simulink model "forces_cosimulation"  (R2021b)
settings: Solver=ode45  StartTime=0.0  StopTime=40  FixedStep=0.01  RelTol=1e-3  EnableMultiTasking=on
libraries: instrumentlib x2, simulink x2
settings Model: PacingRate=11  Creator=tasora  LastModifiedBy=Trevor
settings SolverCC: AlgebraicLoopSolver=TrustRegion
settings DataIOCC: LimitDataPoints=on  SaveFormat=Array  SignalLoggingSaveFormat=ModelDataLogs  ReturnWorkspaceOutputs=off
settings OptimizationCC: ExpressionDepthLimit=2147483647  LifeSpan=inf
settings DebuggingCC: UnderspecifiedInitializationDetection=Classic  MergeDetectMultiDrivingBlocksExec=none  SolverPrmCheckMsg=warning  FcnCallInpInsideContextMsg=warning  StateNameClashWarn=warning  SFUnexpectedBacktrackingDiag=warning  SFNoUnconditionalDefaultTransitionDiag=warning  SFExecutionAtInitializationDiag=none  SFMachineParentedDataDiag=warning  ArithmeticOperatorsInVariantConditions=warning
settings HardwareCC: ProdBitPerPointer=32  ProdBitPerSizeT=32  ProdBitPerPtrDiffT=32  ProdLargestAtomicFloat=None  ProdIntDivRoundTo=Undefined  ProdEndianess=Unspecified  ProdWordSize=32  ProdHWDeviceType=32-bit Generic
settings ModelReferenceCC: PropagateSignalLabelsOutOfModel=off
settings SFSimCC: SimUseLocalCustomCode=off  CustomCodeUndefinedFunction=UseInterfaceOnly
settings RTWCC: RTWUseLocalCustomCode=off
settings CodeAppCC: StateflowObjectComments=on
settings GRTTargetCC: TargetLangStandard=C89/C90 (ANSI)  CombineOutputUpdateFcns=off  GRTInterface=on
settings ConfigComp: CovMetricSettings=dw  CovSaveCumulativeToWorkspaceVar=on  CovSaveSingleToWorkspaceVar=on  CovExternalEMLEnable=off

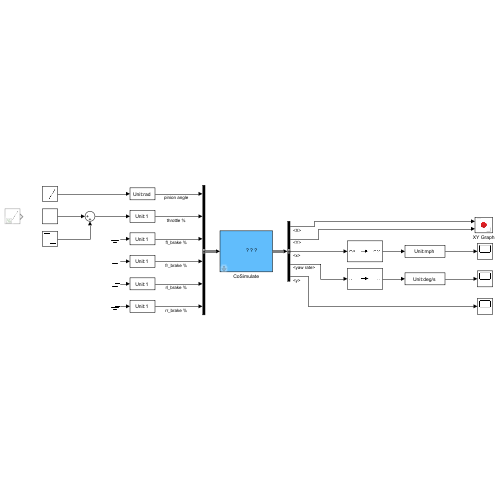
[thumbnail: Simulink's stored preview of the top-level diagram]
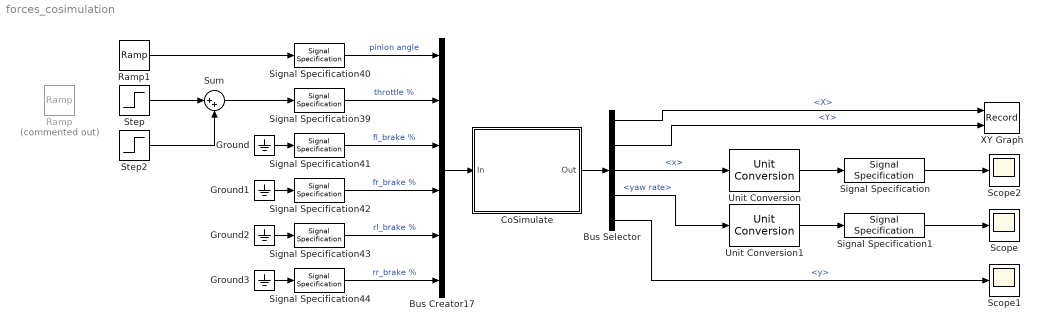
== system forces_cosimulation ==
  Bus Creator17 : BusCreator  Inputs=6
  Bus Selector : BusSelector  OutputSignals=global frame.position.X,global frame.position.Y,chassis frame.velocity.x,chassis frame.rotational velocity.yaw rate,chassis frame.acceleration.y
  CoSimulate : Subsystem  Description=|  mask{com_step=1e-2, tcp_data_size=39, host_name=localhost, tcp_port=50009, tcp_timeout=5}
      | This block can be used to exchange data with Chrono::Engine.                                                                                      
      | A Chrono::Engine program with a running ChCosimulation inferface must be started, it will work as a server; then the Simulink program must be run.
      | Note! check that the dimensions of the exchanged vectors do match!
      mask prompts: com_step "Communication step size"; tcp_data_size "N. of scalars received from C::E (as block output)"; host_name "TCP host name (ex. 'localhost', or 'www.myhost.com')"; tcp_port "TCP port (ex. 50007)"; tcp_timeout "TCP timeout (seconds)"
      mask init:
      | block_receive = [gcb, '/TCP Receive'];
      | set_param(block_receive, 'SampleTime', num2str(com_step));
      | set_param(block_receive, 'Host', host_name);
      | set_param(block_receive, 'Port', num2str(tcp_port));
      | set_param(block_receive, 'DataSize', num2str(tcp_data_size+1));
      | set_param(block_receive, 'Timeout', num2str(tcp_timeout));
      | block_send = [gcb, '/TCP Send'];
      | set_param(block_send, 'Host', host_name);
      | set_param(block_send, 'Port', num2str(tcp_port));
      mask Display:
      | image(imread('block_logo.png'))
      | disp('C::E                   ')
  Ground{,1..3} (4 alike) : Ground
  Ramp : simulink/Sources/Ramp  Commented=on  slope=0.1  start=4  InitialOutput=0
  Ramp1 : simulink/Sources/Ramp  slope=0.01  start=15  InitialOutput=0
  Scope : Scope
  Scope1 : Scope
  Scope2 : Scope
  Signal Specification : SignalSpecification  Unit=mph
  Signal Specification1 : SignalSpecification  Unit=deg/s
  Signal Specification{39,41..44} (5 alike) : SignalSpecification  Unit=1
  Signal Specification40 : SignalSpecification  Unit=rad
  Step : Step  Time=3  After=0.75  SampleTime=0
  Step2 : Step  Time=15  After=-0.05  SampleTime=0
  Sum : Sum  Inputs=|++
  Unit Conversion : UnitConversion
  Unit Conversion1 : UnitConversion
  XY Graph : Record  FileSettingsInternal="{\"entries\":[{\"content\":{\"excelSettings\":{\"content\":{},\"type\":\"Streamout.ExcelSettings\"}},\"type\":\"Streamout.FileSettingStorage\",\"uuid\":\"5bc0685a-b1bb-4583-b74f-d6d04f37d9c6\"}],\"packageUris\":[\"http://schema.mathworks.com/mf0/streamout_blocks/R2020a\"],\"version\":\"1.0\"}"  Layout=[1 1]  SignalsInternal="{\"entries\":[{\"content\":{\"signals\":[{\"content\":{\"blockPath\":[\"forces_cosimulation/XY Graph\"],\"channel\":[],\"dimensions\":[1,1],\"domain\":\"forces_cosimulation/XY Graph\",\"lineColor\":\"#a2142f\",\"plots\":[1],\"port\":1,\"sid\":[\"\"],\"signalID\":3435,\"signalName\":\"<X>\"},\"type\":\"RecordBlkView.Signal\",\"uuid\":\"5aa4ce1d-9ab9-452c-9b58-d05b75f7601c\"},{\"content\":{\"blockPath\":[\"forces_cosimulation/XY Graph\"],\"channel\":[],\"dimensions\":[1,1],\"domain\":\"forces_cosimulation/XY Graph\",\"lineColor\":\"#139fff\",\"plots\":[1],\"port\":2,\"sid\":[\"\"],\"signalID\":3439,\"signalName\":\"<Y>\"},\"type\":\"RecordBlkView.Signal\",\"uuid\":\"38391aed-c002-4d5f-92b2-354e32cfb4eb\"}]},\"type\":\"RecordBlkView.InputSignals\",\"uuid\":\"4796c31f-e78f-4ee8-b460-c380f51b4893\"}],\"packageUris\":[\"http://schema.mathworks.com/mf0/streamout_blocks/R2020a\"],\"version\":\"1.0\"}"  VisualizationBindings="{\"xyplotplugin\":{\"info\":[{\"series\":[{\"bindingParametersList\":[{\"parameter\":\"X-Axis\",\"signalID\":3435,\"signalName\":\"<X>\"},{\"parameter\":\"Y-Axis\",\"signalID\":3439,\"signalName\":\"<Y>\"}],\"seriesID\":12101}],\"subplotID\":1}]}}"  CompatibilityTag=XY
  wires:
  Step/1 -> Sum/1
  Step2/1 -> Sum/2
  Signal Specification44/1 -> Bus Creator17/6  "rr_brake %"
  Signal Specification40/1 -> Bus Creator17/1  "pinion angle"
  Signal Specification39/1 -> Bus Creator17/2  "throttle %"
  Signal Specification42/1 -> Bus Creator17/4  "fr_brake %"
  Signal Specification41/1 -> Bus Creator17/3  "fl_brake %"
  Signal Specification43/1 -> Bus Creator17/5  "rl_brake %"
  Bus Creator17/1 -> CoSimulate/1(In)
  Ramp1/1 -> Signal Specification40/1
  Sum/1 -> Signal Specification39/1
  CoSimulate/1(Out) -> Bus Selector/1
  Bus Selector/1 -> XY Graph/1  "<X>"
  Bus Selector/2 -> XY Graph/2  "<Y>"
  Bus Selector/4 -> Unit Conversion1/1  "<yaw rate>"
  Bus Selector/5 -> Scope1/1  "<y>"
  Ground/1 -> Signal Specification41/1
  Ground1/1 -> Signal Specification42/1
  Ground2/1 -> Signal Specification43/1
  Ground3/1 -> Signal Specification44/1
  Bus Selector/3 -> Unit Conversion/1  "<x>"
  Unit Conversion/1 -> Signal Specification/1
  Signal Specification/1 -> Scope2/1
  Unit Conversion1/1 -> Signal Specification1/1
  Signal Specification1/1 -> Scope/1

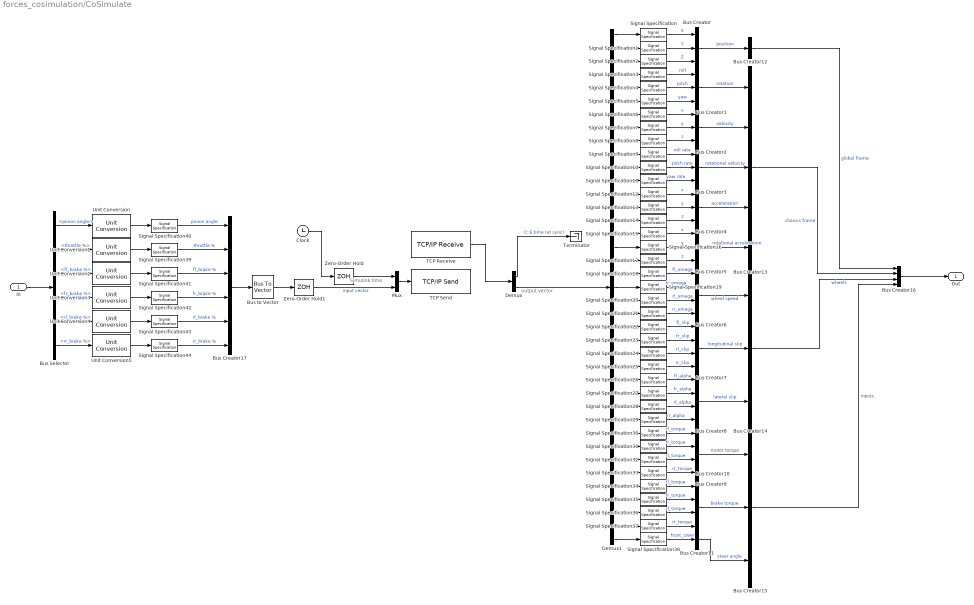
== system forces_cosimulation/CoSimulate ==
  note: output vector
  note: Simulink time
  In : Inport
  Bus Creator{,1..5,14..15} (8 alike) : BusCreator  Inputs=3
  Bus Creator{6..10,16} (6 alike) : BusCreator  Inputs=4
  Bus Creator11 : BusCreator  Inputs=1
  Bus Creator12 : BusCreator  Inputs=1
  Bus Creator13 : BusCreator  Inputs=5
  Bus Creator17 : BusCreator  Inputs=6
  Bus Selector : BusSelector  OutputSignals=pinion angle,throttle %,fl_brake %,fr_brake %,rl_brake %,rr_brake %
  Bus to Vector : BusToVector
  Clock : Clock
  Demux : Demux  Outputs=[1 -1]
  Demux1 : Demux  Outputs=39
  Mux : Mux  Inputs=2
  Signal Specification : SignalSpecification  Unit=m
  Signal Specification1 : SignalSpecification  Unit=m
  Signal Specification{9..11,18..21} (7 alike) : SignalSpecification  Unit=rad/s
  Signal Specification12 : SignalSpecification  Unit=m/s^2
  Signal Specification13 : SignalSpecification  Unit=m/s^2
  Signal Specification14 : SignalSpecification  Unit=m/s^2
  Signal Specification15 : SignalSpecification  Unit=rad/s^2
  Signal Specification16 : SignalSpecification  Unit=rad/s^2
  Signal Specification17 : SignalSpecification  Unit=rad/s^2
  Signal Specification2 : SignalSpecification  Unit=m
  Signal Specification{22..25,39,41..44} (9 alike) : SignalSpecification  Unit=1
  Signal Specification{3..5,26..29,38,40} (9 alike) : SignalSpecification  Unit=rad
  Signal Specification{30..37} (8 alike) : SignalSpecification  Unit=N*m
  Signal Specification6 : SignalSpecification  Unit=m/s
  Signal Specification7 : SignalSpecification  Unit=m/s
  Signal Specification8 : SignalSpecification  Unit=m/s
  TCP Receive : instrumentlib/TCP//IP Receive  Priority=1  Host=localhost  Port=50009  DataSize=40  DataType=double  ASCIIFormatting=%f  Terminator=LF  CustomTerminator=10  ByteOrder=little-endian  EnableBlockingMode=on  Timeout=5  SampleTime=0.01  SimulateUsing=Interpreted execution
  TCP Send : instrumentlib/TCP//IP Send  Priority=2  Host=localhost  Port=50009  ByteOrder=little-endian  EnableBlockingMode=off  Timeout=10  TransferDelay=on  SimulateUsing=Interpreted execution
  Terminator : Terminator
  Unit Conversion{,1..5} (6 alike) : UnitConversion
  Zero-Order Hold : ZeroOrderHold  SampleTime=com_step
  Zero-Order Hold1 : ZeroOrderHold  SampleTime=com_step
  Out : Outport
  wires:
  Zero-Order Hold/1 -> Mux/1
  Zero-Order Hold1/1 -> Mux/2  "input vector"
  Mux/1 -> TCP Send/1
  Clock/1 -> Zero-Order Hold/1
  In/1 -> Bus Selector/1
  TCP Receive/1 -> Demux/1
  Demux/1 -> Terminator/1  "C::E time (at sync)"
  Demux/2 -> Demux1/1
  Demux1/4 -> Signal Specification3/1
  Demux1/1 -> Signal Specification/1
  Demux1/3 -> Signal Specification2/1
  Demux1/10 -> Signal Specification9/1
  Demux1/2 -> Signal Specification1/1
  Demux1/7 -> Signal Specification6/1
  Demux1/11 -> Signal Specification10/1
  Demux1/9 -> Signal Specification8/1
  Demux1/5 -> Signal Specification4/1
  Demux1/6 -> Signal Specification5/1
  Demux1/12 -> Signal Specification11/1
  Demux1/8 -> Signal Specification7/1
  Signal Specification/1 -> Bus Creator/1  "X"
  Signal Specification1/1 -> Bus Creator/2  "Y"
  Signal Specification2/1 -> Bus Creator/3  "Z"
  Signal Specification3/1 -> Bus Creator1/1  "roll"
  Signal Specification4/1 -> Bus Creator1/2  "pitch"
  Signal Specification5/1 -> Bus Creator1/3  "yaw"
  Signal Specification6/1 -> Bus Creator2/1  "x"
  Signal Specification7/1 -> Bus Creator2/2  "y"
  Signal Specification8/1 -> Bus Creator2/3  "z"
  Signal Specification9/1 -> Bus Creator3/1  "roll rate"
  Signal Specification10/1 -> Bus Creator3/2  "pitch rate"
  Signal Specification11/1 -> Bus Creator3/3  "yaw rate"
  Demux1/13 -> Signal Specification12/1
  Demux1/15 -> Signal Specification14/1
  Demux1/14 -> Signal Specification13/1
  Signal Specification12/1 -> Bus Creator4/1  "x"
  Signal Specification13/1 -> Bus Creator4/2  "y"
  Signal Specification14/1 -> Bus Creator4/3  "z"
  Demux1/16 -> Signal Specification15/1
  Demux1/17 -> Signal Specification16/1
  Demux1/18 -> Signal Specification17/1
  Signal Specification15/1 -> Bus Creator5/1  "x"
  Signal Specification16/1 -> Bus Creator5/2  "y"
  Signal Specification17/1 -> Bus Creator5/3  "z"
  Demux1/19 -> Signal Specification18/1
  Demux1/20 -> Signal Specification19/1
  Demux1/21 -> Signal Specification20/1
  Demux1/22 -> Signal Specification21/1
  Signal Specification21/1 -> Bus Creator6/4  "rr_omega"
  Signal Specification20/1 -> Bus Creator6/3  "rl_omega"
  Signal Specification19/1 -> Bus Creator6/2  "fr_omega"
  Signal Specification18/1 -> Bus Creator6/1  "fl_omega"
  Demux1/23 -> Signal Specification22/1
  Demux1/24 -> Signal Specification23/1
  Demux1/26 -> Signal Specification25/1
  Demux1/25 -> Signal Specification24/1
  Signal Specification22/1 -> Bus Creator7/1  "fl_slip"
  Signal Specification23/1 -> Bus Creator7/2  "fr_slip"
  Signal Specification24/1 -> Bus Creator7/3  "rl_slip"
  Signal Specification25/1 -> Bus Creator7/4  "rr_slip"
  Demux1/27 -> Signal Specification26/1
  Demux1/28 -> Signal Specification27/1
  Demux1/29 -> Signal Specification28/1
  Demux1/30 -> Signal Specification29/1
  Signal Specification26/1 -> Bus Creator8/1  "fl_alpha"
  Signal Specification27/1 -> Bus Creator8/2  "fr_alpha"
  Signal Specification28/1 -> Bus Creator8/3  "rl_alpha"
  Signal Specification29/1 -> Bus Creator8/4  "rr_alpha"
  Demux1/31 -> Signal Specification30/1
  Demux1/32 -> Signal Specification31/1
  Demux1/33 -> Signal Specification32/1
  Demux1/34 -> Signal Specification33/1
  Signal Specification30/1 -> Bus Creator9/1  "fl_torque"
  Signal Specification31/1 -> Bus Creator9/2  "fr_torque"
  Signal Specification32/1 -> Bus Creator9/3  "rl_torque"
  Signal Specification33/1 -> Bus Creator9/4  "rr_torque"
  Demux1/35 -> Signal Specification34/1
  Demux1/36 -> Signal Specification35/1
  Demux1/37 -> Signal Specification36/1
  Demux1/38 -> Signal Specification37/1
  Signal Specification34/1 -> Bus Creator10/1  "fl_torque"
  Signal Specification35/1 -> Bus Creator10/2  "fr_torque"
  Signal Specification36/1 -> Bus Creator10/3  "rl_torque"
  Signal Specification37/1 -> Bus Creator10/4  "rr_torque"
  Demux1/39 -> Signal Specification38/1
  Signal Specification38/1 -> Bus Creator11/1  "front_steer"
  Bus Creator/1 -> Bus Creator12/1  "position"
  Bus Creator1/1 -> Bus Creator13/1  "rotation"
  Bus Creator2/1 -> Bus Creator13/2  "velocity"
  Bus Creator3/1 -> Bus Creator13/3  "rotational velocity"
  Bus Creator4/1 -> Bus Creator13/4  "acceleration"
  Bus Creator5/1 -> Bus Creator13/5  "rotational acceleration"
  Bus Creator6/1 -> Bus Creator14/1  "wheel speed"
  Bus Creator7/1 -> Bus Creator14/2  "longitudinal slip"
  Bus Creator8/1 -> Bus Creator14/3  "lateral slip"
  Bus Creator9/1 -> Bus Creator15/1  "motor torque"
  Bus Creator10/1 -> Bus Creator15/2  "brake torque"
  Bus Creator11/1 -> Bus Creator15/3  "steer angle"
  Bus Creator14/1 -> Bus Creator16/3  "wheels"
  Bus Creator15/1 -> Bus Creator16/4  "inputs"
  Bus Creator12/1 -> Bus Creator16/1  "global frame"
  Bus Creator13/1 -> Bus Creator16/2  "chassis frame"
  Bus Creator16/1 -> Out/1
  Bus to Vector/1 -> Zero-Order Hold1/1
  Bus Creator17/1 -> Bus to Vector/1
  Signal Specification40/1 -> Bus Creator17/1  "pinion angle"
  Signal Specification39/1 -> Bus Creator17/2  "throttle %"
  Unit Conversion/1 -> Signal Specification40/1
  Bus Selector/1 -> Unit Conversion/1  "<pinion angle>"
  Unit Conversion1/1 -> Signal Specification39/1
  Unit Conversion2/1 -> Signal Specification41/1
  Unit Conversion4/1 -> Signal Specification43/1
  Unit Conversion5/1 -> Signal Specification44/1
  Unit Conversion3/1 -> Signal Specification42/1
  Signal Specification41/1 -> Bus Creator17/3  "fl_brake %"
  Signal Specification42/1 -> Bus Creator17/4  "fr_brake %"
  Signal Specification43/1 -> Bus Creator17/5  "rl_brake %"
  Signal Specification44/1 -> Bus Creator17/6  "rr_brake %"
  Bus Selector/2 -> Unit Conversion1/1  "<throttle %>"
  Bus Selector/3 -> Unit Conversion2/1  "<fl_brake %>"
  Bus Selector/4 -> Unit Conversion3/1  "<fr_brake %>"
  Bus Selector/5 -> Unit Conversion4/1  "<rl_brake %>"
  Bus Selector/6 -> Unit Conversion5/1  "<rr_brake %>"
